simulink model "ballTossController"  (R2014a)
settings: Solver=FixedStepDiscrete  SolverMode=SingleTasking  StartTime=0.0  StopTime=10.0  FixedStep=dt  RelTol=1e-3
values from neighbouring files (symbols this model uses):
  dt = 0.01    [ballToss.m]
  dtheta1_throw_traj = linspace(0, 1, 10)    [ballToss.m]
  dtheta2_throw_traj = linspace(0, 1, 10)    [ballToss.m]
  Kd1 = 1    [ballToss.m]
  Kd2 = 1    [ballToss.m]
  Kp1 = 180    [ballToss.m]
  Kp2 = 180    [ballToss.m]
  t_ref_init = linspace(0, 1, 10)    [ballToss.m]
  t_ref_throw = linspace(0, 1, 10)    [ballToss.m]
  theta1_init_traj = linspace(0, 1, 10)    [ballToss.m]
  theta1_throw_traj = linspace(0, 1, 10)    [ballToss.m]
  theta2_init_traj = linspace(0, 1, 10)    [ballToss.m]
  theta2_throw_traj = linspace(0, 1, 10)    [ballToss.m]
libraries: cstblocks x4, legonxtlib x4, simulink_extras x2, simulink x2
settings Model: SimulationMode=external  ExtModeTrigDuration=2  Creator=yutongfeng  LastModifiedBy=yutongfeng
settings OptimizationCC: OptimizeModelRefInitCode=on  LifeSpan=1
settings DebuggingCC: UnderspecifiedInitializationDetection=Classic  SolverPrmCheckMsg=none
settings HardwareCC: ProdLargestAtomicInteger=Long  ProdLargestAtomicFloat=Float  ProdEndianess=LittleEndian  ProdHWDeviceType=ARM Compatible->ARM 7
settings RTWCC: SystemTargetFile=realtime.tlc  GenerateMakefile=off  TemplateMakefile=realtime.tmf  Description=Run on Target Hardware  RTWVerbose=off  ProcessScript=realtime_make_rtw_hook
settings STFCustomTargetCC: TargetLibSuffix=.a  GenerateSampleERTMain=on  ConcurrentExecutionCompliant=off  GeneratePreprocessorConditionals=Use local settings  ERTCustomFileBanners=on  SupportNonInlinedSFcns=off  SupportVariableSizeSignals=on  MATLABClassNameForMDSCustomization=Simulink.SoftwareTarget.ERTCustomization  GRTInterface=off  SystemTargetFile=realtime.tlc
settings ERTTargetCC: CombineOutputUpdateFcns=off  SupportContinuousTime=on  SupportVariableSizeSignals=on  ExtModeTransport=2  ExtModeMexFile=ext_serial_win32_comm_no_acks_rtt  ExtModeMexArgs=0 1 9600  ERTSrcFileBannerTemplate=realtime_code_template.cgt  ERTHdrFileBannerTemplate=realtime_code_template.cgt  ERTDataSrcFileTemplate=realtime_code_template.cgt  ERTDataHdrFileTemplate=realtime_code_template.cgt  ERTCustomFileTemplate=realtime_file_process.tlc

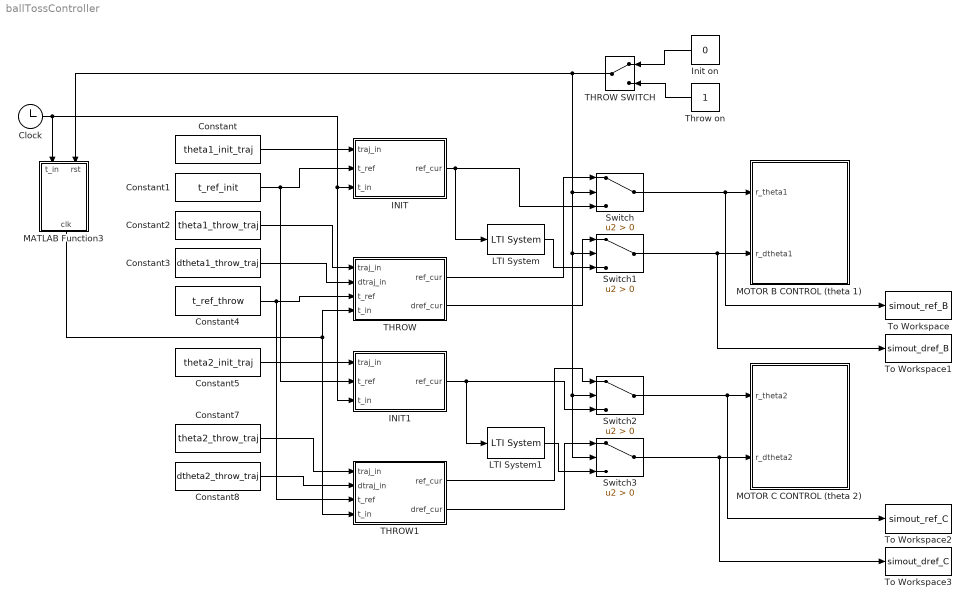
== system ballTossController ==
  Clock : Clock
  Constant : Constant  Value=theta1_init_traj
  Constant1 : Constant  Value=t_ref_init
  Constant2 : Constant  Value=theta1_throw_traj
  Constant3 : Constant  Value=dtheta1_throw_traj
  Constant4 : Constant  Value=t_ref_throw
  Constant5 : Constant  Value=theta2_init_traj
  Constant7 : Constant  Value=theta2_throw_traj
  Constant8 : Constant  Value=dtheta2_throw_traj
  INIT : MATLAB Function  TreatAsAtomicUnit=on
  INIT1 : MATLAB Function  TreatAsAtomicUnit=on
  Init on : Constant  Value=0
  LTI System : cstblocks/LTI System  sys=dttf  IC=[]
  LTI System1 : cstblocks/LTI System  sys=dttf  IC=[]
  MATLAB Function3 : MATLAB Function  TreatAsAtomicUnit=on
  MOTOR B CONTROL (theta 1) : Subsystem
  MOTOR C CONTROL (theta 2) : Subsystem
  Switch{,1..3} (4 alike) : Switch  Criteria=u2 > Threshold
  THROW : MATLAB Function  TreatAsAtomicUnit=on
  THROW SWITCH : ManualSwitch
  THROW1 : MATLAB Function  TreatAsAtomicUnit=on
  Throw on : Constant
  To Workspace : ToWorkspace  VariableName=simout_ref_B  SaveFormat=Structure With Time  SampleTime=-1
  To Workspace1 : ToWorkspace  VariableName=simout_dref_B  SaveFormat=Structure With Time  SampleTime=-1
  To Workspace2 : ToWorkspace  VariableName=simout_ref_C  SaveFormat=Structure With Time  SampleTime=-1
  To Workspace3 : ToWorkspace  VariableName=simout_dref_C  SaveFormat=Structure With Time  SampleTime=-1
  wires:
  Throw on/1 -> THROW SWITCH/2
  Init on/1 -> THROW SWITCH/1
  THROW SWITCH/1 -> MATLAB Function3/2(rst), Switch3/2, Switch2/2, Switch1/2, Switch/2
  Switch1/1 -> To Workspace1/1, MOTOR B CONTROL (theta 1)/2(r_dtheta1)
  Switch/1 -> To Workspace/1, MOTOR B CONTROL (theta 1)/1(r_theta1)
  Switch2/1 -> To Workspace2/1, MOTOR C CONTROL (theta 2)/1(r_theta2)
  Switch3/1 -> MOTOR C CONTROL (theta 2)/2(r_dtheta2), To Workspace3/1
  INIT/1(ref_cur) -> Switch/3, LTI System/1
  THROW/1(ref_cur) -> Switch/1
  Constant/1 -> INIT/1(traj_in)
  Clock/1 -> MATLAB Function3/1(t_in), INIT1/3(t_in), INIT/3(t_in)
  Constant7/1 -> THROW1/1(traj_in)
  Constant8/1 -> THROW1/2(dtraj_in)
  Constant5/1 -> INIT1/1(traj_in)
  INIT1/1(ref_cur) -> LTI System1/1, Switch2/3
  LTI System/1 -> Switch1/3
  LTI System1/1 -> Switch3/3
  THROW/2(dref_cur) -> Switch1/1
  THROW1/1(ref_cur) -> Switch2/1
  THROW1/2(dref_cur) -> Switch3/1
  Constant1/1 -> INIT/2(t_ref), INIT1/2(t_ref)
  MATLAB Function3/1(clk) -> THROW/4(t_in), THROW1/4(t_in)
  Constant2/1 -> THROW/1(traj_in)
  Constant3/1 -> THROW/2(dtraj_in)
  Constant4/1 -> THROW1/3(t_ref), THROW/3(t_ref)

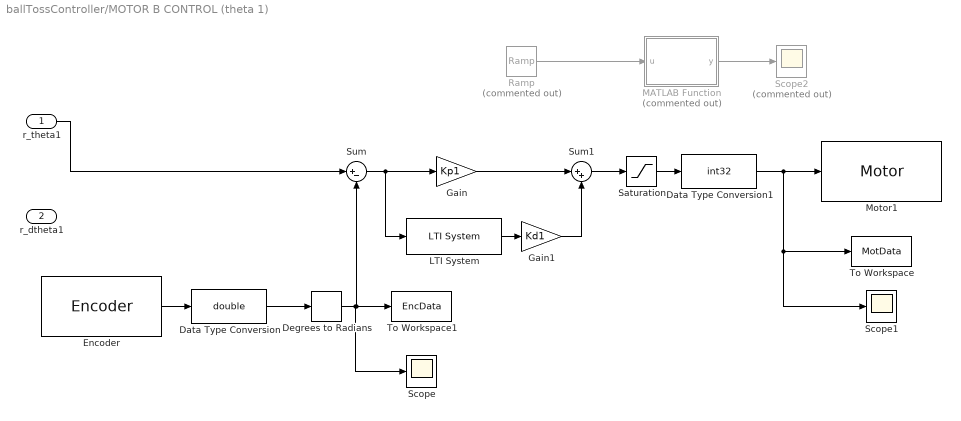
== system ballTossController/MOTOR B CONTROL (theta 1) ==
  r_theta1 : Inport
  r_dtheta1 : Inport  Port=2
  Data Type Conversion : DataTypeConversion  OutMin=-100  OutMax=100  OutDataTypeStr=double
  Data Type Conversion1 : DataTypeConversion  OutMin=-100  OutMax=100  OutDataTypeStr=int32
  Degrees to Radians : simulink_extras/Transformations/Degrees to Radians
  Encoder : legonxtlib/Encoder  portNumber=B  opMode=No reset  sampleTime=dt
  Gain : Gain  Gain=Kp1
  Gain1 : Gain  Gain=Kd1
  LTI System : cstblocks/LTI System  sys=dttf  IC=[]
  MATLAB Function : MATLAB Function  Commented=on  TreatAsAtomicUnit=on
  Motor1 : legonxtlib/Motor  sportNumber=B  sstopAction=Brake
  Ramp : simulink/Sources/Ramp  Commented=on  slope=1  start=0  X0=0
  Saturation : Saturate  UpperLimit=100  LowerLimit=-100  SampleTime=dt
  Scope : Scope
      settings: YMin=-0.5  YMax=6.5
  Scope1 : Scope
      settings: YMin=2.85  YMax=3.15
  Scope2 : Scope  Commented=on
      settings: YMin=0  YMax=30  SaveName=ScopeData2
  Sum : Sum  Inputs=|+-
  Sum1 : Sum  Inputs=|++
  To Workspace : ToWorkspace  VariableName=MotData  SaveFormat=Structure With Time  SampleTime=dt
  To Workspace1 : ToWorkspace  VariableName=EncData  SaveFormat=Structure With Time  SampleTime=dt
  wires:
  Saturation/1 -> Data Type Conversion1/1
  Data Type Conversion/1 -> Degrees to Radians/1
  Degrees to Radians/1 -> To Workspace1/1, Sum/2, Scope/1
  Data Type Conversion1/1 -> Scope1/1, To Workspace/1, Motor1/1
  Encoder/1 -> Data Type Conversion/1
  Sum/1 -> Gain/1, LTI System/1
  Gain/1 -> Sum1/1
  Sum1/1 -> Saturation/1
  Ramp/1 -> MATLAB Function/1(u)
  MATLAB Function/1(y) -> Scope2/1
  r_theta1/1 -> Sum/1
  LTI System/1 -> Gain1/1
  Gain1/1 -> Sum1/2

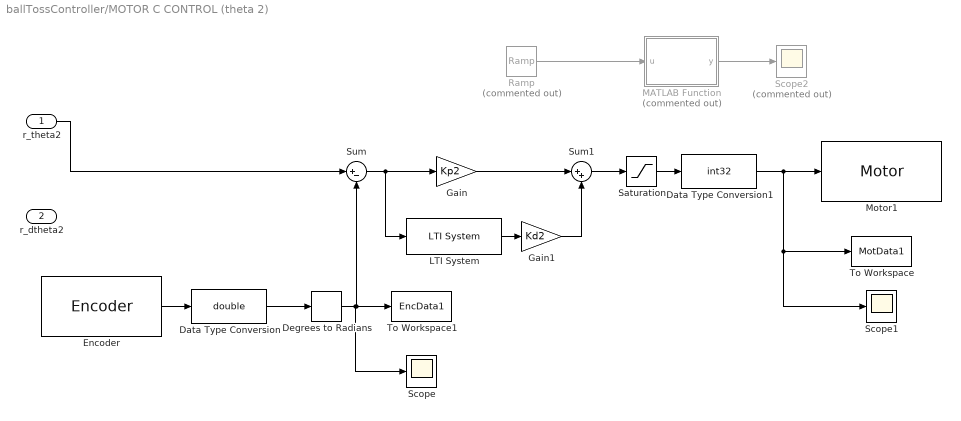
== system ballTossController/MOTOR C CONTROL (theta 2) ==
  r_theta2 : Inport
  r_dtheta2 : Inport  Port=2
  Data Type Conversion : DataTypeConversion  OutMin=-100  OutMax=100  OutDataTypeStr=double
  Data Type Conversion1 : DataTypeConversion  OutMin=-100  OutMax=100  OutDataTypeStr=int32
  Degrees to Radians : simulink_extras/Transformations/Degrees to Radians
  Encoder : legonxtlib/Encoder  portNumber=C  opMode=No reset  sampleTime=dt
  Gain : Gain  Gain=Kp2
  Gain1 : Gain  Gain=Kd2
  LTI System : cstblocks/LTI System  sys=dttf  IC=[]
  MATLAB Function : MATLAB Function  Commented=on  TreatAsAtomicUnit=on
  Motor1 : legonxtlib/Motor  sportNumber=C  sstopAction=Brake
  Ramp : simulink/Sources/Ramp  Commented=on  slope=1  start=0  X0=0
  Saturation : Saturate  UpperLimit=100  LowerLimit=-100  SampleTime=dt
  Scope : Scope
      settings: YMin=-0.5  YMax=6.5  SaveName=ScopeData3
  Scope1 : Scope
      settings: YMin=2.85  YMax=3.15  SaveName=ScopeData4
  Scope2 : Scope  Commented=on
      settings: YMin=0  YMax=30  SaveName=ScopeData5
  Sum : Sum  Inputs=|+-
  Sum1 : Sum  Inputs=|++
  To Workspace : ToWorkspace  VariableName=MotData1  SaveFormat=Structure With Time  SampleTime=dt
  To Workspace1 : ToWorkspace  VariableName=EncData1  SaveFormat=Structure With Time  SampleTime=dt
  wires:
  Saturation/1 -> Data Type Conversion1/1
  Data Type Conversion/1 -> Degrees to Radians/1
  Degrees to Radians/1 -> To Workspace1/1, Sum/2, Scope/1
  Data Type Conversion1/1 -> Scope1/1, To Workspace/1, Motor1/1
  Encoder/1 -> Data Type Conversion/1
  Sum/1 -> Gain/1, LTI System/1
  Gain/1 -> Sum1/1
  Sum1/1 -> Saturation/1
  Ramp/1 -> MATLAB Function/1(u)
  MATLAB Function/1(y) -> Scope2/1
  r_theta2/1 -> Sum/1
  LTI System/1 -> Gain1/1
  Gain1/1 -> Sum1/2

== matlab function ballTossController/INIT ==
  data: traj_in input; t_ref input; ref_cur output; t_in input
function ref_cur = fcn(traj_in, t_ref, t_in)
if t_in < 0
    ref_cur = 0;
elseif t_in > t_ref(end)
    ref_cur = traj_in(end);
else
    ref_cur = interp1(t_ref, traj_in, t_in);
end

== matlab function ballTossController/MOTOR B CONTROL (theta 1)/MATLAB Function ==
  data: u input; y output
function y = fcn(u)
tref = [1 11];
yref = [0 pi];
if u<tref(1)
y = 0;
elseif u>tref(end);
y = yref(end);
else
y = interp1(tref,yref,u);
end

== matlab function ballTossController/THROW ==
  data: traj_in input; dtraj_in input; t_ref input; ref_cur output; t_in input; dref_cur output
function [ref_cur, dref_cur] = fcn(traj_in, dtraj_in, t_ref, t_in)
if t_in < 0
    ref_cur = 0;
    dref_cur = 0;
elseif t_in > t_ref(end)
    ref_cur = traj_in(end);
    dref_cur = dtraj_in(end);
else
    ref_cur = interp1(t_ref, traj_in, t_in);
    dref_cur = interp1(t_ref, dtraj_in, t_in);
end

== matlab function ballTossController/INIT1 ==
  data: traj_in input; t_ref input; ref_cur output; t_in input
function ref_cur = fcn(traj_in, t_ref, t_in)
if t_in < 0
    ref_cur = 0;
elseif t_in > t_ref(end)
    ref_cur = traj_in(end);
else
    ref_cur = interp1(t_ref, traj_in, t_in);
end

== matlab function ballTossController/MATLAB Function3 ==
  data: t_in input; clk output; rst input
function clk = fcn(t_in, rst)
persistent t_off last_rst
if isempty(t_off)
    t_off = 0;
end
if isempty(last_rst)
    last_rst = 0;
end

if abs(rst - last_rst) ~= 0
    t_off = t_in;
end

clk = t_in - t_off;
last_rst = rst;

== matlab function ballTossController/THROW1 ==
  data: traj_in input; dtraj_in input; t_ref input; ref_cur output; t_in input; dref_cur output
function [ref_cur, dref_cur] = fcn(traj_in, dtraj_in, t_ref, t_in)
if t_in < 0
    ref_cur = 0;
    dref_cur = 0;
elseif t_in > t_ref(end)
    ref_cur = traj_in(end);
    dref_cur = dtraj_in(end);
else
    ref_cur = interp1(t_ref, traj_in, t_in);
    dref_cur = interp1(t_ref, dtraj_in, t_in);
end

== matlab function ballTossController/MOTOR C CONTROL (theta 2)/MATLAB Function ==
  data: u input; y output
function y = fcn(u)
tref = [1 11];
yref = [0 pi];
if u<tref(1)
y = 0;
elseif u>tref(end);
y = yref(end);
else
y = interp1(tref,yref,u);
end
